simulink model "time_gongji_KVHpost"  (R2019b)
settings: Solver=ode3  StartTime=0.0  StopTime=6000  FixedStep=0.01  MaxStep=0.01  RelTol=1e-3
values from neighbouring files (symbols this model uses):
  bias_gyro_z_gongji = -0.7e-3    (= -0.0007)    [sych_ite_KVHpost_daoyuan_huace.m]
settings Model: Creator=luyishi_E480  LastModifiedBy=xie_z
settings DataIOCC: SaveOutput=off  SignalLogging=off  DSMLogging=off  InspectSignalLogs=on  SaveTime=off  ReturnWorkspaceOutputs=off
settings DebuggingCC: InheritedTsInSrcMsg=none

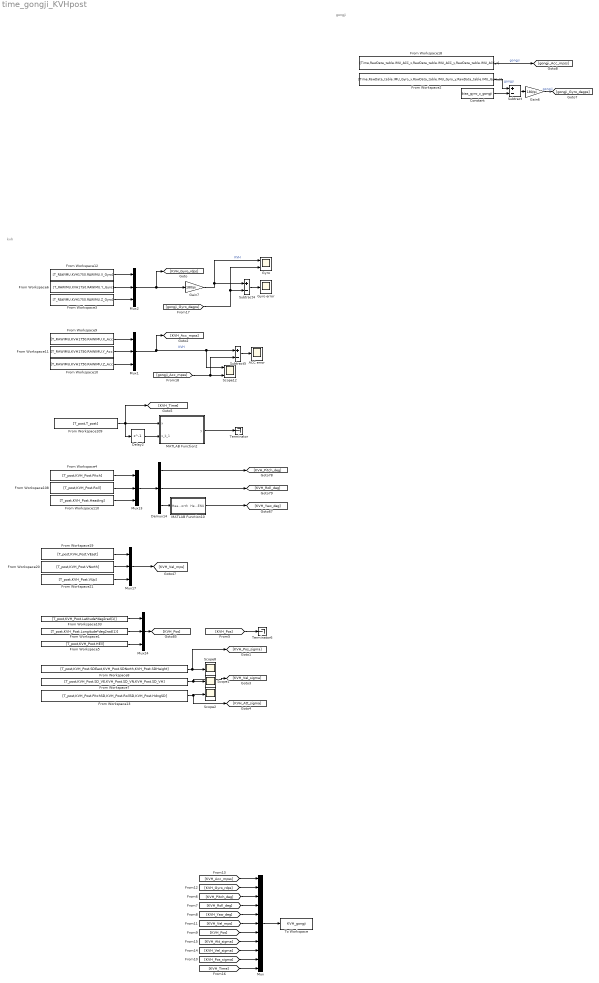
== system time_gongji_KVHpost ==
  note: gongji
  note: kvh
  ACC error : Scope
  Constant : Constant  Value=bias_gyro_z_gongji
  Delay2 : Delay  DelayLength=1  InitialCondition=0
  Demux14 : Demux  Outputs=3
  From Workspace1 : FromWorkspace  VariableName=[T_post,KVH_Post.Longitude*deg2rad(1)]  OutputAfterFinalValue=Holding final value
  From Workspace10 : FromWorkspace  VariableName=[T_RAWIMU,KVH1750.RAWIMU.Z_Acc]  Interpolate=off  OutputAfterFinalValue=Holding final value
  From Workspace103 : FromWorkspace  VariableName=[T_post,KVH_Post.Latitude*deg2rad(1)]  OutputAfterFinalValue=Holding final value
  From Workspace108 : FromWorkspace  VariableName=[T_post,KVH_Post.Roll]  Interpolate=off  OutputAfterFinalValue=Holding final value
  From Workspace109 : FromWorkspace  VariableName=[T_post,T_post]  Interpolate=off  OutputAfterFinalValue=Holding final value
  From Workspace11 : FromWorkspace  VariableName=[T_RAWIMU,KVH1750.RAWIMU.Y_Acc]  Interpolate=off  OutputAfterFinalValue=Holding final value
  From Workspace110 : FromWorkspace  VariableName=[T_post,KVH_Post.Heading]  Interpolate=off  OutputAfterFinalValue=Holding final value
  From Workspace12 : FromWorkspace  VariableName=[T_RAWIMU,KVH1750.RAWIMU.X_Gyro]  Interpolate=off  OutputAfterFinalValue=Holding final value
  From Workspace13 : FromWorkspace  VariableName=[T_post,KVH_Post.PitchSD,KVH_Post.RollSD,KVH_Post.HdngSD]  Interpolate=off  OutputAfterFinalValue=Holding final value
  From Workspace18 : FromWorkspace  VariableName=[Time,RawData_table.IMU_ACC_x,RawData_table.IMU_ACC_y,RawData_table.IMU_ACC_z]  Interpolate=off  OutputAfterFinalValue=Holding final value
  From Workspace19 : FromWorkspace  VariableName=[T_post,KVH_Post.VEast]  Interpolate=off  OutputAfterFinalValue=Holding final value
  From Workspace2 : FromWorkspace  VariableName=[Time,RawData_table.IMU_Gyro_x,RawData_table.IMU_Gyro_y,RawData_table.IMU_Gyro_z]  Interpolate=off  OutputAfterFinalValue=Holding final value
  From Workspace20 : FromWorkspace  VariableName=[T_post,KVH_Post.VNorth]  Interpolate=off  OutputAfterFinalValue=Holding final value
  From Workspace21 : FromWorkspace  VariableName=[T_post,KVH_Post.VUp]  Interpolate=off  OutputAfterFinalValue=Holding final value
  From Workspace3 : FromWorkspace  VariableName=[T_RAWIMU,KVH1750.RAWIMU.Z_Gyro]  Interpolate=off  OutputAfterFinalValue=Holding final value
  From Workspace4 : FromWorkspace  VariableName=[T_post,KVH_Post.Pitch]  Interpolate=off  OutputAfterFinalValue=Holding final value
  From Workspace5 : FromWorkspace  VariableName=[T_post,KVH_Post.HEll]  OutputAfterFinalValue=Holding final value
  From Workspace6 : FromWorkspace  VariableName=[T_RAWIMU,KVH1750.RAWIMU.Y_Gyro]  Interpolate=off  OutputAfterFinalValue=Holding final value
  From Workspace7 : FromWorkspace  VariableName=[T_post,KVH_Post.SD_VE,KVH_Post.SD_VN,KVH_Post.SD_VH]  Interpolate=off  OutputAfterFinalValue=Holding final value
  From Workspace8 : FromWorkspace  VariableName=[T_post,KVH_Post.SDEast,KVH_Post.SDNorth,KVH_Post.SDHeight]  Interpolate=off  OutputAfterFinalValue=Holding final value
  From Workspace9 : FromWorkspace  VariableName=[T_RAWIMU,KVH1750.RAWIMU.X_Acc]  Interpolate=off  OutputAfterFinalValue=Holding final value
  Gain6 : Gain  Gain=180/pi
  Gain7 : Gain  Gain=180/pi
  "Gyro " : Scope  NumInputPorts=2
  Gyro error : Scope
  MATLAB Function10 : MATLAB Function  TreatAsAtomicUnit=on
  MATLAB Function2 : MATLAB Function  TreatAsAtomicUnit=on
  Mux : Mux  Inputs=11
  Mux{1..2,13,17,24} (5 alike) : Mux  Inputs=3
  Scope1 : Scope
  Scope12 : Scope  NumInputPorts=2
  Scope2 : Scope
  Scope8 : Scope
  Subtract : Sum  Inputs=+-
  Subtract4 : Sum  Inputs=+-
  Subtract5 : Sum  Inputs=+-
  Terminator : Terminator
  Terminator6 : Terminator
  To Workspace : ToWorkspace  VariableName=KVH_gongji  SaveFormat=Structure With Time  SampleTime=-1
  wires:
  Delay2/1 -> MATLAB Function2/2(x_k_1)
  From Workspace109/1 -> [KVH_Time], Delay2/1, MATLAB Function2/1(x)
  MATLAB Function2/1(y) -> Terminator/1
  Mux2/1 -> [KVH_Gyro_rdps], Gain7/1
  Subtract4/1 -> Gyro error/1
  Subtract5/1 -> ACC error/1
  Gain7/1 -> "Gyro "/1, Subtract4/1  "KVH"
  Mux1/1 -> [KVH_Acc_mpss], Subtract5/1, Scope12/1  "KVH"
  From Workspace110/1 -> Mux13/3
  Demux14/1 -> [KVH_Pitch_deg]
  MATLAB Function10/1(Heading_ENU) -> [KVH_Yaw_deg]
  Mux13/1 -> Demux14/1
  Demux14/2 -> [KVH_Roll_deg]
  From Workspace108/1 -> Mux13/2
  From Workspace4/1 -> Mux13/1
  Demux14/3 -> MATLAB Function10/1(Heading_North)
  From Workspace20/1 -> Mux17/2
  From Workspace21/1 -> Mux17/3
  From Workspace19/1 -> Mux17/1
  Mux17/1 -> [KVH_Vel_mps]
  Mux24/1 -> [KVH_Pos]
  From Workspace103/1 -> Mux24/1
  From Workspace5/1 -> Mux24/3
  From Workspace1/1 -> Mux24/2
  From Workspace8/1 -> [KVH_Pos_sigma], Scope8/1
  From Workspace9/1 -> Mux1/1
  From Workspace11/1 -> Mux1/2
  From Workspace10/1 -> Mux1/3
  From Workspace3/1 -> Mux2/3
  From Workspace6/1 -> Mux2/2
  From Workspace12/1 -> Mux2/1
  [KVH_Pos] -> Terminator6/1
  [KVH_Pitch_deg] -> Mux/3
  [KVH_Roll_deg] -> Mux/4
  [KVH_Acc_mpss] -> Mux/1
  [KVH_Gyro_rdps] -> Mux/2
  [KVH_Yaw_deg] -> Mux/5
  [KVH_Vel_mps] -> Mux/6
  [KVH_Pos] -> Mux/7
  Mux/1 -> To Workspace/1
  From Workspace7/1 -> [KVH_Vel_sigma], Scope1/1
  From Workspace13/1 -> Scope2/1, [KVH_Att_sigma]
  [KVH_Att_sigma] -> Mux/8
  [KVH_Vel_sigma] -> Mux/9
  [KVH_Pos_sigma] -> Mux/10
  [KVH_Time] -> Mux/11
  Subtract/1 -> Gain6/1
  Constant/1 -> Subtract/2
  From Workspace2/1 -> Subtract/1  "gongji"
  From Workspace18/1 -> [gongji_Acc_mpss]  "gongji"
  Gain6/1 -> [gongji_Gyro_degps]  "gongji"
  [gongji_Gyro_degps] -> Subtract4/2, "Gyro "/2
  [gongji_Acc_mpss] -> Subtract5/2, Scope12/2

== matlab function time_gongji_KVHpost/MATLAB Function2 ==
  data: y output; x input; x_k_1 input
function y  = fcn(x,x_k_1)
    if x ~= x_k_1
        y = uint8(1);
    else
        y = uint8(0);
    end
end

== matlab function time_gongji_KVHpost/MATLAB Function10 ==
  data: Heading_North input; Heading_ENU output size=1
function Heading_ENU = fcn(Heading_North)
% Heading_ENU:以北为零顺时针为正0-360°
% Heading_North:以北为零逆时针为正-180-180°

% Heading_North = Heading_North + 0.5 + 3.8;
if Heading_North <= 180
    Heading_ENU = 0 - Heading_North;
else
    Heading_ENU = 360 - Heading_North;
end
